simulink model "reverb"  (R2016a)
settings: Solver=VariableStepAuto  StartTime=0.0  StopTime=10.0  RelTol=1e-3
libraries: dspsrcs4 x1
settings Model: Creator=joa-m  LastModifiedBy=joa-m

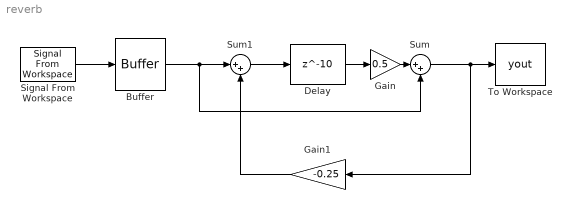
== system reverb ==
  Buffer : Buffer  N=1  TreatMby1Signals=One channel  OutputFrames=off
  Delay : Delay  DelayLength=10  InputProcessing=Columns as channels (frame based)
  Gain : Gain  Gain=0.5
  Gain1 : Gain  Gain=-0.25
  Signal From Workspace : dspsrcs4/Signal From Workspace  X=[0,0.125,0.25,0.5,0.75,0,0,0]  Ts=1  nsamps=1  OutputAfterFinalValue=Setting to zero  ignoreOrWarnInputAndFrameLengths=off  OutputFrames=off
  Sum : Sum  Inputs=|++
  Sum1 : Sum  Inputs=|++
  To Workspace : ToWorkspace  VariableName=yout  SampleTime=-1
      settings: Save2DSignal=2-D array (concatenate along first dimension)
  wires:
  Sum1/1 -> Delay/1
  Buffer/1 -> Sum/2, Sum1/1
  Signal From Workspace/1 -> Buffer/1
  Delay/1 -> Gain/1
  Gain/1 -> Sum/1
  Gain1/1 -> Sum1/2
  Sum/1 -> Gain1/1, To Workspace/1
